simulink model "deadtime_compensation"  (R2022a)
settings: Solver=FixedStepAuto  StartTime=0.0  StopTime=10.0  RelTol=1e-3
PostLoadFcn:
  | , if any(exist('dsrtsu_mdlpostloadfcn', 'file') == [2, 3, 6]), try dsrtsu_mdlpostloadfcn('Execute', bdroot); catch fprintf('Error in PostLoadFcn (dsrtsu_mdlpostloadfcn) for model "%s":\n %s\n', bdroot, lasterr); end, end,
undefined symbols (not defined in the file): dead_time, fpwm
settings Model: DSRTSU_INTERNAL_RTI_VER=510  DSRTSU_INTERNAL_RTI_TYPE=rti1202  RTICANMMDATA=struct('GeneralSetupData',struct('modelroot','C:\Users\z634594\Documents\MATLAB\Projects\powerHIL\reference','generalsettings',struct('filesettings',struct('destfolder',struct('Name','RTICANMM_FILES','Check',1),'buildfolder',struct('Name','.','Check',1),'AbsDestfolder',struct('Name','C:\Users\z634594\Documents\MATLAB\Projects\powerHIL\reference\RTICANMM_FILES'),'AbsBuildfolder',struct('Name','C:\Users\z634594\Documents\MATLAB\Projects\powerHIL\reference'))),'options',struct('addpaths',1,'rmpaths',1,'addtrcexclusion',logical(1),'cannavigator',struct('checkmonitoring',0),'show_usrtrc',0,'use_usrtrc',0),'advanced',struct('options',[1 1 1 1 1 1 1 1 1 1 1 1 1 1 1 1 1 1 1 1 1 1 1 1 1 1 1 1 1 1 1 1 1 1 1 1 1 1 1 1 1 1 1 1 1 1 1 1 1 1 1 1 1 1 1 1 1 1 1 1 1 1 1 1 1 1 1 1 1 1 1 1 1 1 1 1 1 1 1 1 1 1 1 1 1 1 1 1 1 1 1 1 1 1 1 1 1 1 1 1]),'MPSetup',{{}},'modelname','deadtime_compensation','block','deadtime_compensation'))  DSRTSU_INTERNAL_RTIFLEXRAYCONFIG=110  Creator=Z634594  LastModifiedBy=z634594
settings SolverCC: AlgebraicLoopSolver=TrustRegion
settings DataIOCC: ReturnWorkspaceOutputs=off
settings DebuggingCC: UnconnectedInputMsg=warning  UnconnectedOutputMsg=warning  UnconnectedLineMsg=warning  SFMachineParentedDataDiag=warning  ArithmeticOperatorsInVariantConditions=warning
settings HardwareCC: ProdBitPerPointer=32  ProdBitPerSizeT=32  ProdBitPerPtrDiffT=32  ProdLargestAtomicInteger=Integer  ProdEndianess=BigEndian  ProdWordSize=32  ProdHWDeviceType=Custom Processor->Custom  TargetIntDivRoundTo=Zero  TargetEndianess=BigEndian  TargetHWDeviceType=Custom Processor->Custom
settings SFSimCC: SimUseLocalCustomCode=off  MATLABDynamicMemAlloc=off  CustomCodeUndefinedFunction=UseInterfaceOnly
settings RTWCC: Description=dSPACE DS1202 Hardware Platform  SystemTargetFile=rti1202.tlc  MakeCommand=make_rti  TemplateMakefile=rti1202.tmf  RTWUseLocalCustomCode=off  DLArmComputeVersion=19.05
settings STFCustomTargetCC: ParMdlRefBuildCompliant=on  MatFileLogging=on  GRTInterface=off  SystemTargetFile=rti1202.tlc
settings GRTTargetCC: TargetLangStandard=C89/C90 (ANSI)  CompOptLevelCompliant=off  ConcurrentExecutionCompliant=off  CombineOutputUpdateFcns=off  CPPClassGenCompliant=off  UseToolchainInfoCompliant=off

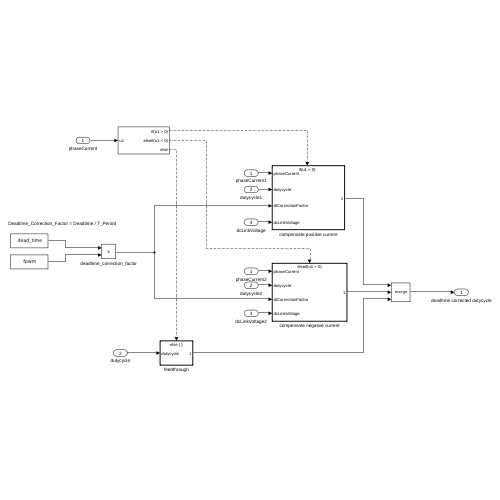
[thumbnail: Simulink's stored preview of the top-level diagram]
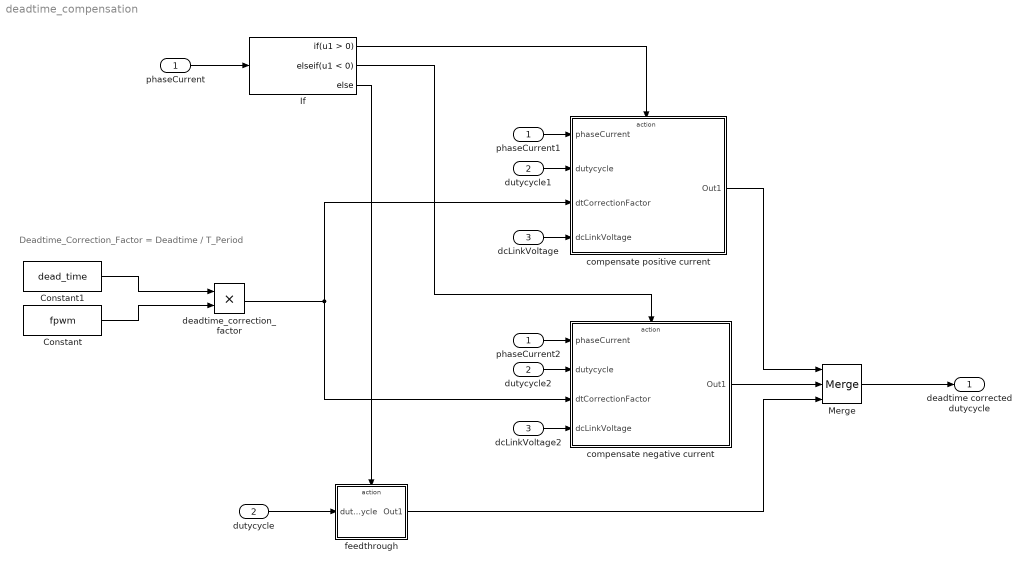
== system deadtime_compensation ==
  note: Deadtime_Correction_Factor = Deadtime / T_Period
  phaseCurrent : Inport
  dutycycle : Inport  Port=2
  dcLinkVoltage : Inport  Port=3
  Constant : Constant  Value=fpwm
  Constant1 : Constant  Value=dead_time
  If : If  ElseIfExpressions=u1 < 0
  Merge : Merge  Inputs=3
  compensate negative current : Subsystem  TreatAsAtomicUnit=on
  compensate positive current : Subsystem  TreatAsAtomicUnit=on
  dcLinkVoltage2 : InportShadow  Port=3
  deadtime_correction_factor : Product
  dutycycle1 : InportShadow  Port=2
  dutycycle2 : InportShadow  Port=2
  feedthrough : Subsystem  TreatAsAtomicUnit=on
  phaseCurrent1 : InportShadow
  phaseCurrent2 : InportShadow
  deadtime corrected dutycycle : Outport  VectorParamsAs1DForOutWhenUnconnected=off
  wires:
  deadtime_correction_factor/1 -> compensate positive current/3(dtCorrectionFactor), compensate negative current/3(dtCorrectionFactor)
  phaseCurrent/1 -> If/1
  If/3 -> feedthrough/Action
  dutycycle1/1 -> compensate positive current/2(dutycycle)
  If/2 -> compensate negative current/Action
  Constant1/1 -> deadtime_correction_factor/1
  Constant/1 -> deadtime_correction_factor/2
  phaseCurrent1/1 -> compensate positive current/1(phaseCurrent)
  dutycycle/1 -> feedthrough/1(dutycycle)
  Merge/1 -> deadtime corrected dutycycle/1
  feedthrough/1(Out1) -> Merge/3
  phaseCurrent2/1 -> compensate negative current/1(phaseCurrent)
  compensate negative current/1(Out1) -> Merge/2
  If/1 -> compensate positive current/Action
  compensate positive current/1(Out1) -> Merge/1
  dutycycle2/1 -> compensate negative current/2(dutycycle)
  dcLinkVoltage/1 -> compensate positive current/4(dcLinkVoltage)
  dcLinkVoltage2/1 -> compensate negative current/4(dcLinkVoltage)

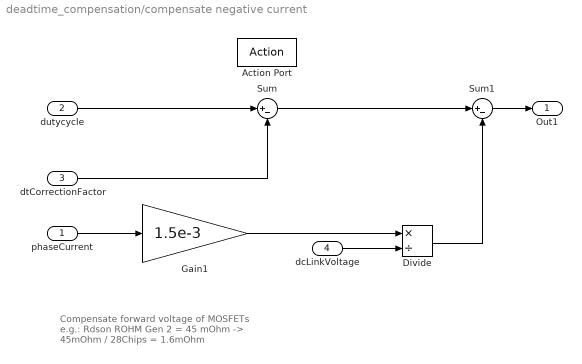
== system deadtime_compensation/compensate negative current ==
  note: Compensate forward voltage of MOSFETs
      | e.g.: Rdson ROHM Gen 2 = 45 mOhm
      | -> 45mOhm / 28Chips = 1.6mOhm
  phaseCurrent : Inport
  dutycycle : Inport  Port=2
  dtCorrectionFactor : Inport  Port=3
  dcLinkVoltage : Inport  Port=4
  Action Port : ActionPort  ActionPortLabel=elseif(u1 < 0)
  Divide : Product  Inputs=*/
  Gain1 : Gain  Gain=1.5e-3
  Sum : Sum  Inputs=|+-
  Sum1 : Sum  Inputs=|+-
  Out1 : Outport  VectorParamsAs1DForOutWhenUnconnected=off
  wires:
  dutycycle/1 -> Sum/1
  phaseCurrent/1 -> Gain1/1
  Sum/1 -> Sum1/1
  Sum1/1 -> Out1/1
  dtCorrectionFactor/1 -> Sum/2
  Gain1/1 -> Divide/1
  Divide/1 -> Sum1/2
  dcLinkVoltage/1 -> Divide/2

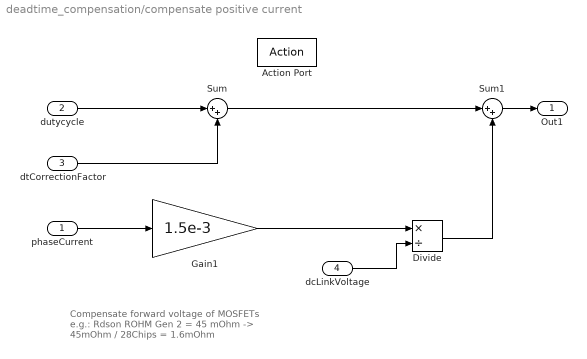
== system deadtime_compensation/compensate positive current ==
  note: Compensate forward voltage of MOSFETs
      | e.g.: Rdson ROHM Gen 2 = 45 mOhm
      | -> 45mOhm / 28Chips = 1.6mOhm
  phaseCurrent : Inport
  dutycycle : Inport  Port=2
  dtCorrectionFactor : Inport  Port=3
  dcLinkVoltage : Inport  Port=4
  Action Port : ActionPort  ActionPortLabel=if(u1 > 0)
  Divide : Product  Inputs=*/
  Gain1 : Gain  Gain=1.5e-3
  Sum : Sum  Inputs=|++
  Sum1 : Sum  Inputs=|++
  Out1 : Outport  VectorParamsAs1DForOutWhenUnconnected=off
  wires:
  dutycycle/1 -> Sum/1
  Sum/1 -> Sum1/1
  Sum1/1 -> Out1/1
  dtCorrectionFactor/1 -> Sum/2
  Gain1/1 -> Divide/1
  Divide/1 -> Sum1/2
  phaseCurrent/1 -> Gain1/1
  dcLinkVoltage/1 -> Divide/2

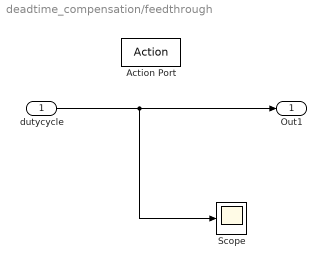
== system deadtime_compensation/feedthrough ==
  dutycycle : Inport
  Action Port : ActionPort  ActionPortLabel=else
  Scope : Scope
  Out1 : Outport  VectorParamsAs1DForOutWhenUnconnected=off
  wires:
  dutycycle/1 -> Scope/1, Out1/1
